simulink model "node23_case_10kV_withLoad_v2"  (R2022b)
settings: Solver=VariableStepAuto  StartTime=0.0  StopTime=10  FixedStep=1e-6  RelTol=1e-5
InitFcn:
  | sw=5;
  | Lf=1.75e-3+3.5e-3;
  | %Lf=3.5e-3;
  | %Cf=2e-4;
  | f=10;
  | Cf=15e-6;
  | % L=1.75e-3/2;
  | % X=100*pi*L;
  | % R=2*X;
  | R=0.25;X=R/0.66;
  | L=X/100/pi;
  | Z=sqrt(R^2+X^2);
  | f = 30;
  | kp1=10;
  | ki1=100;
  | kp4=20;
  | ki4=100;
  | kp16=20;
  | ki16=100;
  | % 负载参数
  | R1L=0;
  | X1L=0;
  | R2L=652.4467;
  | X2L=276.0351;
  | R3L=804.5741;
  | X3L=256.7790;
  | R4L=760.9867;
  | X4L=234.6376;
  | R5L=818.7384;
  | X5L=266.9799;
  | R6L=671.1329;
  | X6L=170.1801;
  | R7L=883.7621;
  | X7L=178.8663;
  | R8L=388.3725;
  | X8L=158.3040;
  | R9L=817.4819;
  | X9L=268.6933;
  | R10L=849.4733;
  | X10L=254.8420;
  | R11L=407.8415;
  | X11L=165.8504;
  | R12L=NaN;  % Bus 12 无 R、X 数据，用 NaN 标记
  | X12L=NaN;
  | R13L=751.2339;
  | X13L=329.8428;
  | R14L=294.0393;
  | X14L=141.6929;
  | R15L=761.9027;
  | X15L=284.3908;
  | R16L=740.4040;
  | X16L=318.2438;
  | R17L=674.5784;
  | X17L=316.4689;
  | R18L=776.7449;
  | X18L=316.6080;
  | R19L=766.0423;
  | X19L=335.7994;
  | R20L=746.0545;
  | X20L=344.3329;
  | R21L=706.9418;
  | X21L=357.8658;
  | R22L=702.3905;
  | X22L=304.8773;
  | R23L=244.5696;
  | X23L=118.4449;
  | %% Case 1
  | % I4dp_ref = 68.7653;
  | % I4qp_ref = -94.1021;
  | % I4dn_ref = 39.6776;
  | % I4qn_ref = -27.1728;
  | % I8dp_ref = 68.5903;
  | % I8qp_ref = -93.5945;
  | % I8dn_ref = 40.6189;
  | % I8qn_ref = -26.6634;
  | % I10dp_ref = 62.5266;
  | % I10qp_ref = -85.5137;
  | % I10dn_ref = 42.9996;
  | % I10qn_ref = -28.7612;
  | % I11dp_ref = 62.7521;
  | % I11qp_ref = -85.7827;
  | % I11dn_ref = 42.8345;
  | % I11qn_ref = -28.6532;
  | % I12dp_ref = 62.3475;
  | % I12qp_ref = -85.2997;
  | % I12dn_ref = 43.1344;
  | % I12qn_ref = -28.848;
  | % I16dp_ref = 82.4934;
  | % I16qp_ref = -110.4734;
  | % I16dn_ref = 40.1418;
  | % I16qn_ref = -24.7044;
  | % I21dp_ref = 73.1603;
  | % I21qp_ref = -97.1416;
  | % I21dn_ref = 45.9939;
  | % I21qn_ref = -31.0997;
  | % I22dp_ref = 80.0535;
  | % I22qp_ref = -107.1896;
  | % I22dn_ref = 40.9482;
  | % I22qn_ref = -26.0625;
  | % I23dp_ref = 75.9498;
  | % I23qp_ref = -101.1053;
  | % I23dn_ref = 43.7688;
  | % I23qn_ref = -29.0712;
  | %% Case1 comparison 1
  | % I4dp_ref = 111.7874;
  | % I4qp_ref = -170.7915;
  | % I4dn_ref = 0;
  | % I4qn_ref = 0;
  | % I8dp_ref = 52.2536;
  | % I8qp_ref = -33.9901;
  | % I8dn_ref = 0;
  | % I8qn_ref = 0;
  | % I10dp_ref = 33.1037;
  | % I10qp_ref = -19.0499;
  | % I10dn_ref = 0;
  | % I10qn_ref = 0;
  | % I11dp_ref = 43.6215;
  | % I11qp_ref = -22.5412;
  | % I11dn_ref = 0;
  | % I11qn_ref = 0;
  | % I12dp_ref = 8.2667;
  | % I12qp_ref = -27.5019;
  | % I12dn_ref = 0;
  | % I12qn_ref = 0;
  | % I16dp_ref = 104.5239;
  | % I16qp_ref = -104.5004;
  | % I16dn_ref = 0;
  | % I16qn_ref = 0;
  | % I21dp_ref = 68.3072;
  | % I21qp_ref = 6.327;
  | % I21dn_ref = 0;
  | % I21qn_ref = 0;
  | % I22dp_ref = 124.4645;
  | % I22qp_ref = -71.238;
  | % I22dn_ref = 0;
  | % I22qn_ref = 0;
  | % I23dp_ref = -36.8953;
  | % I23qp_ref = -101.2509;
  | % I23dn_ref = 0;
  | % I23qn_ref = 0;
  | 
  | % %%case 1 S2
  | % I4dp_ref = 0;
  | % I4qp_ref = 0;
  | % I4dn_ref = 42.8306;
  | % I4qn_ref = 0;
  | % I8dp_ref = 0;
  | % I8qp_ref = 0;
  | % I8dn_ref = 0;
  | % I8qn_ref = -148.8111;
  | % I10dp_ref = 0;
  | % I10qp_ref = 0;
  | % I10dn_ref = 204.1241;
  | % I10qn_ref = 0;
  | % I11dp_ref = 0;
  | % I11qp_ref = 0;
  | % I11dn_ref = 0;
  | % I11qn_ref = -7.0259;
  | % I12dp_ref = 0;
  | % I12qp_ref = 0;
  | % I12dn_ref = 59.8066;
  | % I12qn_ref = 0;
  | % I16dp_ref = 0;
  | % I16qp_ref = 0;
  | % I16dn_ref = 0;
  | % I16qn_ref = 40.0795;
  | % I21dp_ref = 0;
  | % I21qp_ref = 0;
  | % I21dn_ref = 133.7305;
  | % I21qn_ref = 41.6572;
  | % I22dp_ref = 0;
  | % I22qp_ref = 0;
  | % I22dn_ref = 0;
  | % I22qn_ref = 0;
  | % I23dp_ref = 0;
  | % I23qp_ref = 0;
  | % I23dn_ref = 0;
  | % I23qn_ref = -141.9369;
  | %% Case 2
  | % I4dp_ref = 59.2929;
  | % I4qp_ref = -107.5927;
  | % I4dn_ref = -11.6305;
  | % I4qn_ref = -80.5926;
  | % I8dp_ref = 59.4332;
  | % I8qp_ref = -112.5957;
  | % I8dn_ref = -13.993;
  | % I8qn_ref = -80.1364;
  | % I10dp_ref = 58.9639;
  | % I10qp_ref = -112.9937;
  | % I10dn_ref = -14.0895;
  | % I10qn_ref = -80.4774;
  | % I11dp_ref = 59.0086;
  | % I11qp_ref = -112.9917;
  | % I11dn_ref = -14.1006;
  | % I11qn_ref = -80.4455;
  | % I12dp_ref = 58.9134;
  | % I12qp_ref = -112.9993;
  | % I12dn_ref = -14.0713;
  | % I12qn_ref = -80.5073;
  | % I16dp_ref = 60.7969;
  | % I16qp_ref = -109.8449;
  | % I16dn_ref = -12.6646;
  | % I16qn_ref = -78.7002;
  | % I21dp_ref = 61.3666;
  | % I21qp_ref = -114.9373;
  | % I21dn_ref = -14.6537;
  | % I21qn_ref = -77.5067;
  | % I22dp_ref = 61.0222;
  | % I22qp_ref = -111.4137;
  | % I22dn_ref = -13.2536;
  | % I22qn_ref = -78.3425;
  | % I23dp_ref = 61.4875;
  | % I23qp_ref = -114.3173;
  | % I23dn_ref = -14.4491;
  | % I23qn_ref = -77.5307;
  | 
  | %% case 2 S1
  | % I4dp_ref = 112.192;
  | % I4qp_ref = -170.5275;
  | % I4dn_ref = 0;
  | % I4qn_ref = 0;
  | % I8dp_ref = 112.2722;
  | % I8qp_ref = -170.4747;
  | % I8dn_ref = 0;
  | % I8qn_ref = 0;
  | % I10dp_ref = 111.9451;
  | % I10qp_ref = -170.6897;
  | % I10dn_ref = 0;
  | % I10qn_ref = 0;
  | % I11dp_ref = 111.9882;
  | % I11qp_ref = -170.6614;
  | % I11dn_ref = 0;
  | % I11qn_ref = 0;
  | % I12dp_ref = 111.8926;
  | % I12qp_ref = -170.7241;
  | % I12dn_ref = 0;
  | % I12qn_ref = 0;
  | % I16dp_ref = 112.3621;
  | % I16qp_ref = -170.4154;
  | % I16dn_ref = 0;
  | % I16qn_ref = 0;
  | % I21dp_ref = 112.3273;
  | % I21qp_ref = -170.4384;
  | % I21dn_ref = 0;
  | % I21qn_ref = 0;
  | % I22dp_ref = 112.3902;
  | % I22qp_ref = -170.3969;
  | % I22dn_ref = 0;
  | % I22qn_ref = 0;
  | % I23dp_ref = 112.4817;
  | % I23qp_ref = -170.3365;
  | % I23dn_ref = 0;
  | % I23qn_ref = 0;
  | %% case 2 S2
  | % I4dp_ref = 0;
  | % I4qp_ref = 0;
  | % I4dn_ref = 69.83;
  | % I4qn_ref = -191.8084;
  | % I8dp_ref = 0;
  | % I8qp_ref = 0;
  | % I8dn_ref = -20.269;
  | % I8qn_ref = -203.1153;
  | % I10dp_ref = 0;
  | % I10qp_ref = 0;
  | % I10dn_ref = -45.3511;
  | % I10qn_ref = -199.0225;
  | % I11dp_ref = 0;
  | % I11qp_ref = 0;
  | % I11dn_ref = -12.4369;
  | % I11qn_ref = -203.7449;
  | % I12dp_ref = 0;
  | % I12qp_ref = 0;
  | % I12dn_ref = -12.1733;
  | % I12qn_ref = -203.7608;
  | % I16dp_ref = 0;
  | % I16qp_ref = 0;
  | % I16dn_ref = 48.8908;
  | % I16qn_ref = -198.1826;
  | % I21dp_ref = 0;
  | % I21qp_ref = 0;
  | % I21dn_ref = -43.073;
  | % I21qn_ref = -199.5279;
  | % I22dp_ref = 0;
  | % I22qp_ref = 0;
  | % I22dn_ref = 39.4057;
  | % I22qn_ref = -200.2844;
  | % I23dp_ref = 0;
  | % I23qp_ref = 0;
  | % I23dn_ref = -19.2428;
  | % I23qn_ref = -203.2151;
  | I4dp_ref = 0.9372;
  | I4qp_ref = -0.47047;
  | I4dn_ref = 170.1426;
  | I4qn_ref = -111.8156;
  | I8dp_ref = 28.4579;
  | I8qp_ref = -127.0294;
  | I8dn_ref = 23.3009;
  | I8qn_ref = -14.8212;
  | I10dp_ref = 27.4288;
  | I10qp_ref = -127.8154;
  | I10dn_ref = 16.0506;
  | I10qn_ref = -10.7004;
  | I11dp_ref = 27.4818;
  | I11qp_ref = -127.8231;
  | I11dn_ref = 15.959;
  | I11qn_ref = -10.8247;
  | I12dp_ref = 27.4417;
  | I12qp_ref = -127.7991;
  | I12dn_ref = 16.0832;
  | I12qn_ref = -10.7612;
  | I16dp_ref = 30.7964;
  | I16qp_ref = -47.2674;
  | I16dn_ref = 97.2786;
  | I16qn_ref = -63.7105;
  | I21dp_ref = 33.4859;
  | I21qp_ref = -81.6358;
  | I21dn_ref = 15.3458;
  | I21qn_ref = -5.5591;
  | I22dp_ref = 31.8848;
  | I22qp_ref = -57.1916;
  | I22dn_ref = 83.6176;
  | I22qn_ref = -53.4829;
  | I23dp_ref = 33.8327;
  | I23qp_ref = -82.3263;
  | I23dn_ref = 11.5111;
  | I23qn_ref = -14.1008;
libraries: spsSeriesRLCBranchLib x210, slpidlib x45, spsControlledVoltageSourceLib x30, spsThreePhaseVIMeasurementLib x24, spsPower3phInstantaneousLib x13, spsAlphaBetaZerotoabcLib x9, spsCurrentMeasurementLib x6, spsGroundLib x2, spspowerguiLib x1
(part 1 of 8)
settings Model: SimulationMode=rapid-accelerator  Creator=15224  LastModifiedBy=Sweet_J
settings SolverCC: AlgebraicLoopSolver=TrustRegion
settings DataIOCC: ReturnWorkspaceOutputs=off
settings DebuggingCC: UnconnectedInputMsg=warning  UnconnectedOutputMsg=warning  UnconnectedLineMsg=warning  SFMachineParentedDataDiag=warning  ArithmeticOperatorsInVariantConditions=warning
settings ModelReferenceCC: EnableRefExpFcnMdlSchedulingChecks=on
settings SFSimCC: CustomCodeUndefinedFunction=UseInterfaceOnly

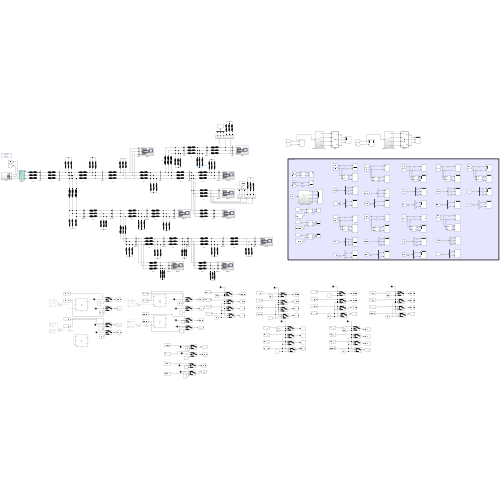
[thumbnail: Simulink's stored preview of the top-level diagram]
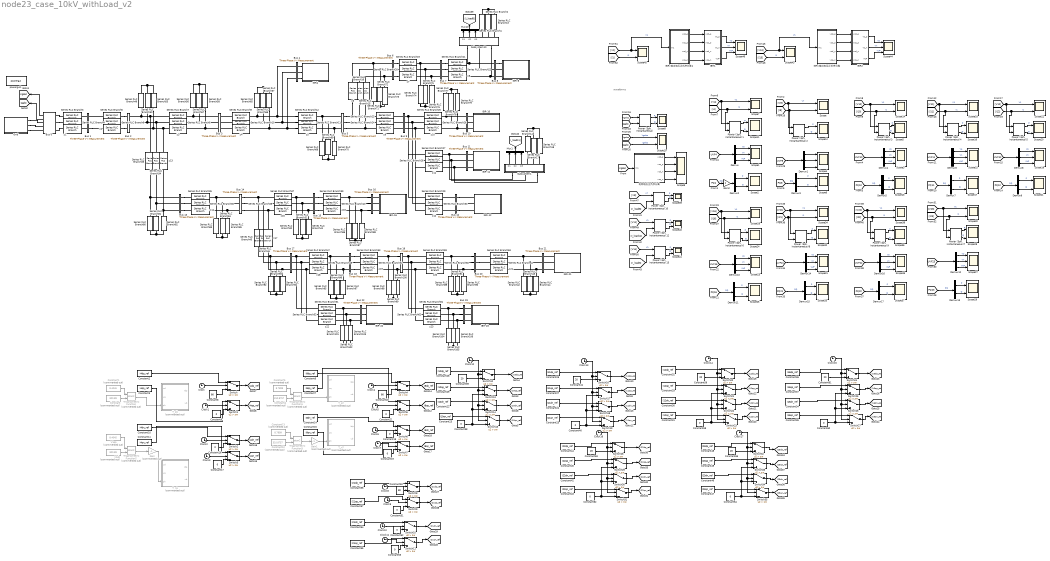
== system node23_case_10kV_withLoad_v2 ==
  note: waveforms
  Bus 0 : spsThreePhaseVIMeasurementLib/Three-Phase V-I Measurement  VoltageMeasurement=phase-to-ground  SetLabelV=off  LabelV=Vabc  Vpu=off  VpuLL=off  CurrentMeasurement=yes  SetLabelI=off  LabelI=Iabc  Ipu=off  Pbase=100e6  Vbase=500e3  OutputType=Complex  PhasorSimulation=off  PSBequivalent=0
  Bus 1 : spsThreePhaseVIMeasurementLib/Three-Phase V-I Measurement  VoltageMeasurement=phase-to-ground  SetLabelV=on  LabelV=V1  Vpu=off  VpuLL=off  CurrentMeasurement=yes  SetLabelI=on  LabelI=I1  Ipu=off  Pbase=100e6  Vbase=500e3  OutputType=Complex  PhasorSimulation=off  PSBequivalent=0
  Bus 10 : spsThreePhaseVIMeasurementLib/Three-Phase V-I Measurement  VoltageMeasurement=phase-to-ground  SetLabelV=on  LabelV=V10  Vpu=off  VpuLL=off  CurrentMeasurement=yes  SetLabelI=on  LabelI=I10  Ipu=off  Pbase=100e6  Vbase=500e3  OutputType=Complex  PhasorSimulation=off  PSBequivalent=0
  Bus 11 : spsThreePhaseVIMeasurementLib/Three-Phase V-I Measurement  VoltageMeasurement=phase-to-ground  SetLabelV=on  LabelV=V11  Vpu=off  VpuLL=off  CurrentMeasurement=yes  SetLabelI=on  LabelI=I11  Ipu=off  Pbase=100e6  Vbase=500e3  OutputType=Complex  PhasorSimulation=off  PSBequivalent=0
  Bus 12 : spsThreePhaseVIMeasurementLib/Three-Phase V-I Measurement  VoltageMeasurement=phase-to-ground  SetLabelV=on  LabelV=V12  Vpu=off  VpuLL=off  CurrentMeasurement=yes  SetLabelI=on  LabelI=I12  Ipu=off  Pbase=100e6  Vbase=500e3  OutputType=Complex  PhasorSimulation=off  PSBequivalent=0
  Bus 13 : spsThreePhaseVIMeasurementLib/Three-Phase V-I Measurement  VoltageMeasurement=phase-to-ground  SetLabelV=on  LabelV=V13  Vpu=off  VpuLL=off  CurrentMeasurement=yes  SetLabelI=on  LabelI=I13  Ipu=off  Pbase=100e6  Vbase=500e3  OutputType=Complex  PhasorSimulation=off  PSBequivalent=0
  Bus 14 : spsThreePhaseVIMeasurementLib/Three-Phase V-I Measurement  VoltageMeasurement=phase-to-ground  SetLabelV=on  LabelV=V14  Vpu=off  VpuLL=off  CurrentMeasurement=yes  SetLabelI=on  LabelI=I14  Ipu=off  Pbase=100e6  Vbase=500e3  OutputType=Complex  PhasorSimulation=off  PSBequivalent=0
  Bus 15 : spsThreePhaseVIMeasurementLib/Three-Phase V-I Measurement  VoltageMeasurement=phase-to-ground  SetLabelV=on  LabelV=V15  Vpu=off  VpuLL=off  CurrentMeasurement=yes  SetLabelI=on  LabelI=I15  Ipu=off  Pbase=100e6  Vbase=500e3  OutputType=Complex  PhasorSimulation=off  PSBequivalent=0
  Bus 16 : spsThreePhaseVIMeasurementLib/Three-Phase V-I Measurement  VoltageMeasurement=phase-to-ground  SetLabelV=on  LabelV=V16  Vpu=off  VpuLL=off  CurrentMeasurement=yes  SetLabelI=on  LabelI=I16  Ipu=off  Pbase=100e6  Vbase=500e3  OutputType=Complex  PhasorSimulation=off  PSBequivalent=0
  Bus 17 : spsThreePhaseVIMeasurementLib/Three-Phase V-I Measurement  VoltageMeasurement=phase-to-ground  SetLabelV=on  LabelV=V17  Vpu=off  VpuLL=off  CurrentMeasurement=yes  SetLabelI=on  LabelI=I17  Ipu=off  Pbase=100e6  Vbase=500e3  OutputType=Complex  PhasorSimulation=off  PSBequivalent=0
  Bus 18 : spsThreePhaseVIMeasurementLib/Three-Phase V-I Measurement  VoltageMeasurement=phase-to-ground  SetLabelV=on  LabelV=V18  Vpu=off  VpuLL=off  CurrentMeasurement=yes  SetLabelI=on  LabelI=I18  Ipu=off  Pbase=100e6  Vbase=500e3  OutputType=Complex  PhasorSimulation=off  PSBequivalent=0
  Bus 19 : spsThreePhaseVIMeasurementLib/Three-Phase V-I Measurement  VoltageMeasurement=phase-to-ground  SetLabelV=on  LabelV=V19  Vpu=off  VpuLL=off  CurrentMeasurement=yes  SetLabelI=on  LabelI=I19  Ipu=off  Pbase=100e6  Vbase=500e3  OutputType=Complex  PhasorSimulation=off  PSBequivalent=0
  Bus 2 : spsThreePhaseVIMeasurementLib/Three-Phase V-I Measurement  VoltageMeasurement=phase-to-ground  SetLabelV=on  LabelV=V2  Vpu=off  VpuLL=off  CurrentMeasurement=yes  SetLabelI=on  LabelI=I2  Ipu=off  Pbase=100e6  Vbase=500e3  OutputType=Complex  PhasorSimulation=off  PSBequivalent=0
  Bus 20 : spsThreePhaseVIMeasurementLib/Three-Phase V-I Measurement  VoltageMeasurement=phase-to-ground  SetLabelV=on  LabelV=V20  Vpu=off  VpuLL=off  CurrentMeasurement=yes  SetLabelI=on  LabelI=I20  Ipu=off  Pbase=100e6  Vbase=500e3  OutputType=Complex  PhasorSimulation=off  PSBequivalent=0
  Bus 21 : spsThreePhaseVIMeasurementLib/Three-Phase V-I Measurement  VoltageMeasurement=phase-to-ground  SetLabelV=on  LabelV=V21  Vpu=off  VpuLL=off  CurrentMeasurement=yes  SetLabelI=on  LabelI=I21  Ipu=off  Pbase=100e6  Vbase=500e3  OutputType=Complex  PhasorSimulation=off  PSBequivalent=0
  Bus 22 : spsThreePhaseVIMeasurementLib/Three-Phase V-I Measurement  VoltageMeasurement=phase-to-ground  SetLabelV=on  LabelV=V22  Vpu=off  VpuLL=off  CurrentMeasurement=yes  SetLabelI=on  LabelI=I22  Ipu=off  Pbase=100e6  Vbase=500e3  OutputType=Complex  PhasorSimulation=off  PSBequivalent=0
  Bus 23 : spsThreePhaseVIMeasurementLib/Three-Phase V-I Measurement  VoltageMeasurement=phase-to-ground  SetLabelV=on  LabelV=V23  Vpu=off  VpuLL=off  CurrentMeasurement=yes  SetLabelI=on  LabelI=I23  Ipu=off  Pbase=100e6  Vbase=500e3  OutputType=Complex  PhasorSimulation=off  PSBequivalent=0
  Bus 3 : spsThreePhaseVIMeasurementLib/Three-Phase V-I Measurement  VoltageMeasurement=phase-to-ground  SetLabelV=on  LabelV=V3  Vpu=off  VpuLL=off  CurrentMeasurement=yes  SetLabelI=on  LabelI=I3  Ipu=off  Pbase=100e6  Vbase=500e3  OutputType=Complex  PhasorSimulation=off  PSBequivalent=0
  Bus 4 : spsThreePhaseVIMeasurementLib/Three-Phase V-I Measurement  VoltageMeasurement=phase-to-ground  SetLabelV=on  LabelV=V4  Vpu=off  VpuLL=off  CurrentMeasurement=yes  SetLabelI=on  LabelI=I4  Ipu=off  Pbase=100e6  Vbase=500e3  OutputType=Complex  PhasorSimulation=off  PSBequivalent=0
  Bus 5 : spsThreePhaseVIMeasurementLib/Three-Phase V-I Measurement  VoltageMeasurement=phase-to-ground  SetLabelV=on  LabelV=V5  Vpu=off  VpuLL=off  CurrentMeasurement=yes  SetLabelI=on  LabelI=I5  Ipu=off  Pbase=100e6  Vbase=500e3  OutputType=Complex  PhasorSimulation=off  PSBequivalent=0
  Bus 6 : spsThreePhaseVIMeasurementLib/Three-Phase V-I Measurement  VoltageMeasurement=phase-to-ground  SetLabelV=on  LabelV=V6  Vpu=off  VpuLL=off  CurrentMeasurement=yes  SetLabelI=on  LabelI=I6  Ipu=off  Pbase=100e6  Vbase=500e3  OutputType=Complex  PhasorSimulation=off  PSBequivalent=0
  Bus 7 : spsThreePhaseVIMeasurementLib/Three-Phase V-I Measurement  VoltageMeasurement=phase-to-ground  SetLabelV=on  LabelV=V7  Vpu=off  VpuLL=off  CurrentMeasurement=yes  SetLabelI=on  LabelI=I7  Ipu=off  Pbase=100e6  Vbase=500e3  OutputType=Complex  PhasorSimulation=off  PSBequivalent=0
  Bus 8 : spsThreePhaseVIMeasurementLib/Three-Phase V-I Measurement  VoltageMeasurement=phase-to-ground  SetLabelV=on  LabelV=V8  Vpu=off  VpuLL=off  CurrentMeasurement=yes  SetLabelI=on  LabelI=I8  Ipu=off  Pbase=100e6  Vbase=500e3  OutputType=Complex  PhasorSimulation=off  PSBequivalent=0
  Bus 9 : spsThreePhaseVIMeasurementLib/Three-Phase V-I Measurement  VoltageMeasurement=phase-to-ground  SetLabelV=on  LabelV=V9  Vpu=off  VpuLL=off  CurrentMeasurement=yes  SetLabelI=on  LabelI=I9  Ipu=off  Pbase=100e6  Vbase=500e3  OutputType=Complex  PhasorSimulation=off  PSBequivalent=0
  Clock{,1..17} (18 alike) : Clock
  Constant : Constant  Commented=on  Value=300.89
  Constant1 : Constant  Commented=on  Value=8.4045
  Constant10 : Constant  Value=I4dn_ref
  Constant11 : Constant  Value=I4qn_ref
  Constant12 : Constant  Commented=on  Value=310.8757
  Constant13 : Constant  Commented=on  Value=8.7899
  Constant14 : Constant  Value=I8dn_ref
  Constant15 : Constant  Value=I8qn_ref
  Constant{9,16..19,21,38,40,51..53,58,60,62,64} (15 alike) : Constant  Value=0
  Constant2 : Constant  Value=I4dp_ref
  Constant20 : Constant  Value=80
  Constant22 : Constant  Value=I10dn_ref
  Constant23 : Constant  Value=I10qn_ref
  Constant24 : Constant  Value=I11dn_ref
  Constant25 : Constant  Value=I11qn_ref
  Constant26 : Constant  Value=I11dp_ref
  Constant27 : Constant  Value=I11qp_ref
  Constant28 : Constant  Value=I10dp_ref
  Constant29 : Constant  Value=I10qp_ref
  Constant3 : Constant  Value=I4qp_ref
  Constant30 : Constant  Value=I12dn_ref
  Constant31 : Constant  Value=I12qn_ref
  Constant32 : Constant  Value=I12dp_ref
  Constant33 : Constant  Value=I12qp_ref
  Constant34 : Constant  Value=I16dn_ref
  Constant35 : Constant  Value=I16qn_ref
  Constant36 : Constant  Value=I16dp_ref
  Constant37 : Constant  Value=I16qp_ref
  Constant{39,41,59,61,63,65} (6 alike) : Constant  Value=20
  Constant4 : Constant  Commented=on  Value=310.8757
  Constant42 : Constant  Value=I22dn_ref
  Constant43 : Constant  Value=I22qn_ref
  Constant44 : Constant  Value=I22dp_ref
  Constant45 : Constant  Value=I22qp_ref
  Constant46 : Constant  Value=I23dn_ref
  Constant47 : Constant  Value=I23qn_ref
  Constant48 : Constant  Value=I23dp_ref
  Constant49 : Constant  Value=I23qp_ref
  Constant5 : Constant  Commented=on  Value=8.7899
  Constant50 : Constant  Value=80
  Constant54 : Constant  Value=I21dn_ref
  Constant55 : Constant  Value=I21qn_ref
  Constant56 : Constant  Value=I21dp_ref
  Constant57 : Constant  Value=I21qp_ref
  Constant6 : Constant  Value=I8dp_ref
  Constant7 : Constant  Value=I8qp_ref
  Constant8 : Constant  Value=80
  Demux{,1,4,6,8,10,12,14,16} (9 alike) : Demux  Outputs=3
  Demux{2..3,5,7,9,11,13,15,17} (9 alike) : Demux  Outputs=2
  Gain : Gain  Commented=on  Gain=-1
  Gain1 : Gain  Commented=on  Gain=-1
  Gain2 : Gain
  Grid : Subsystem
  IBR-10 : Subsystem
  IBR-11 : Subsystem
  IBR-12 : Subsystem
  IBR-16 : Subsystem
  IBR-21 : Subsystem
  IBR-22 : Subsystem
  IBR-23 : Subsystem
  IBR-8 : Subsystem
  IBR1 : MATLAB Function  TreatAsAtomicUnit=on
  IBR1输出电压正负序分离 : Subsystem
  IBR1输出电压正负序分离1 : Subsystem
  IBR2 : MATLAB Function  TreatAsAtomicUnit=on
  IBR4 : Subsystem
  Mux1 : Mux  Inputs=3
  Mux10 : Mux  Inputs=3
  Power (3ph, Instantaneous){,1..10,12..13} (13 alike) : spsPower3phInstantaneousLib/Power (3ph, Instantaneous)
  Scope{,2,5..8,10..14,16..18,20..22,24..26,28..30,32..34,36..41,43,45} (34 alike) : Scope  NumInputPorts=2
  Scope{1,3..4,15,19,23,27,31,35,44,46} (11 alike) : Scope  NumInputPorts=3
  Scope9 : Scope  NumInputPorts=4
  Series RLC Branch1 : spsSeriesRLCBranchLib/Series RLC Branch  LConnTagsString=__new0  RConnTagsString=__new0  BranchType=RL  Resistance=R8L  Inductance=X8L/100/pi  SetiL0=off  InitialCurrent=0  Capacitance=1e-6  Setx0=off  InitialVoltage=0  Measurements=None
  Series RLC Branch{3..12,15..16,19..30,33..40,45..48,51..54,59..64} (46 alike) : spsSeriesRLCBranchLib/Series RLC Branch  LConnTagsString=__new0  RConnTagsString=__new0  BranchType=RL  Resistance=R  Inductance=L  SetiL0=off  InitialCurrent=0  Capacitance=1e-6  Setx0=off  InitialVoltage=0  Measurements=None
  Series RLC Branch100 : spsSeriesRLCBranchLib/Series RLC Branch  LConnTagsString=__new0  RConnTagsString=__new0  BranchType=RL  Resistance=R19L  Inductance=X19L/100/pi  SetiL0=off  InitialCurrent=0  Capacitance=1e-6  Setx0=off  InitialVoltage=0  Measurements=None
  Series RLC Branch101 : spsSeriesRLCBranchLib/Series RLC Branch  LConnTagsString=__new0  RConnTagsString=__new0  BranchType=RL  Resistance=R22L  Inductance=X22L/100/pi  SetiL0=off  InitialCurrent=0  Capacitance=1e-6  Setx0=off  InitialVoltage=0  Measurements=None
  Series RLC Branch102 : spsSeriesRLCBranchLib/Series RLC Branch  LConnTagsString=__new0  RConnTagsString=__new0  BranchType=RL  Resistance=R22L  Inductance=X22L/100/pi  SetiL0=off  InitialCurrent=0  Capacitance=1e-6  Setx0=off  InitialVoltage=0  Measurements=None
  Series RLC Branch103 : spsSeriesRLCBranchLib/Series RLC Branch  LConnTagsString=__new0  RConnTagsString=__new0  BranchType=RL  Resistance=R22L  Inductance=X22L/100/pi  SetiL0=off  InitialCurrent=0  Capacitance=1e-6  Setx0=off  InitialVoltage=0  Measurements=None
  Series RLC Branch104 : spsSeriesRLCBranchLib/Series RLC Branch  LConnTagsString=__new0  RConnTagsString=__new0  BranchType=RL  Resistance=R23L  Inductance=X23L/100/pi  SetiL0=off  InitialCurrent=0  Capacitance=1e-6  Setx0=off  InitialVoltage=0  Measurements=None
  Series RLC Branch105 : spsSeriesRLCBranchLib/Series RLC Branch  LConnTagsString=__new0  RConnTagsString=__new0  BranchType=RL  Resistance=R23L  Inductance=X23L/100/pi  SetiL0=off  InitialCurrent=0  Capacitance=1e-6  Setx0=off  InitialVoltage=0  Measurements=None
  Series RLC Branch106 : spsSeriesRLCBranchLib/Series RLC Branch  LConnTagsString=__new0  RConnTagsString=__new0  BranchType=RL  Resistance=R23L  Inductance=X23L/100/pi  SetiL0=off  InitialCurrent=0  Capacitance=1e-6  Setx0=off  InitialVoltage=0  Measurements=None
  Series RLC Branch13 : spsSeriesRLCBranchLib/Series RLC Branch  LConnTagsString=__new0  RConnTagsString=__new0  BranchType=RL  Resistance=R8L  Inductance=X8L/100/pi  SetiL0=off  InitialCurrent=0  Capacitance=1e-6  Setx0=off  InitialVoltage=0  Measurements=None
  Series RLC Branch14 : spsSeriesRLCBranchLib/Series RLC Branch  LConnTagsString=__new0  RConnTagsString=__new0  BranchType=RL  Resistance=R11L  Inductance=X11L/100/pi  SetiL0=off  InitialCurrent=0  Capacitance=1e-6  Setx0=off  InitialVoltage=0  Measurements=None
  Series RLC Branch17 : spsSeriesRLCBranchLib/Series RLC Branch  LConnTagsString=__new0  RConnTagsString=__new0  BranchType=RL  Resistance=R11L  Inductance=X11L/100/pi  SetiL0=off  InitialCurrent=0  Capacitance=1e-6  Setx0=off  InitialVoltage=0  Measurements=None
  Series RLC Branch18 : spsSeriesRLCBranchLib/Series RLC Branch  LConnTagsString=__new0  RConnTagsString=__new0  BranchType=RL  Resistance=R11L  Inductance=X11L/100/pi  SetiL0=off  InitialCurrent=0  Capacitance=1e-6  Setx0=off  InitialVoltage=0  Measurements=None
  Series RLC Branch2 : spsSeriesRLCBranchLib/Series RLC Branch  LConnTagsString=__new0  RConnTagsString=__new0  BranchType=RL  Resistance=R8L  Inductance=X8L/100/pi  SetiL0=off  InitialCurrent=0  Capacitance=1e-6  Setx0=off  InitialVoltage=0  Measurements=None
  Series RLC Branch31 : spsSeriesRLCBranchLib/Series RLC Branch  LConnTagsString=__new0  RConnTagsString=__new0  BranchType=RL  Resistance=R15L  Inductance=X15L/100/pi  SetiL0=off  InitialCurrent=0  Capacitance=1e-6  Setx0=off  InitialVoltage=0  Measurements=None
  Series RLC Branch32 : spsSeriesRLCBranchLib/Series RLC Branch  LConnTagsString=__new0  RConnTagsString=__new0  BranchType=RL  Resistance=R15L  Inductance=X15L/100/pi  SetiL0=off  InitialCurrent=0  Capacitance=1e-6  Setx0=off  InitialVoltage=0  Measurements=None
  Series RLC Branch41 : spsSeriesRLCBranchLib/Series RLC Branch  LConnTagsString=__new0  RConnTagsString=__new0  BranchType=RL  Resistance=R15L  Inductance=X15L/100/pi  SetiL0=off  InitialCurrent=0  Capacitance=1e-6  Setx0=off  InitialVoltage=0  Measurements=None
  Series RLC Branch42 : spsSeriesRLCBranchLib/Series RLC Branch  LConnTagsString=__new0  RConnTagsString=__new0  BranchType=RL  Resistance=R21L  Inductance=X21L/100/pi  SetiL0=off  InitialCurrent=0  Capacitance=1e-6  Setx0=off  InitialVoltage=0  Measurements=None
  Series RLC Branch43 : spsSeriesRLCBranchLib/Series RLC Branch  LConnTagsString=__new0  RConnTagsString=__new0  BranchType=RL  Resistance=R21L  Inductance=X21L/100/pi  SetiL0=off  InitialCurrent=0  Capacitance=1e-6  Setx0=off  InitialVoltage=0  Measurements=None
  Series RLC Branch44 : spsSeriesRLCBranchLib/Series RLC Branch  LConnTagsString=__new0  RConnTagsString=__new0  BranchType=RL  Resistance=R21L  Inductance=X21L/100/pi  SetiL0=off  InitialCurrent=0  Capacitance=1e-6  Setx0=off  InitialVoltage=0  Measurements=None
  Series RLC Branch49 : spsSeriesRLCBranchLib/Series RLC Branch  LConnTagsString=__new0  RConnTagsString=__new0  BranchType=RL  Resistance=R2L  Inductance=X2L/100/pi  SetiL0=off  InitialCurrent=0  Capacitance=1e-6  Setx0=off  InitialVoltage=0  Measurements=None
  Series RLC Branch50 : spsSeriesRLCBranchLib/Series RLC Branch  LConnTagsString=__new0  RConnTagsString=__new0  BranchType=RL  Resistance=R2L  Inductance=X2L/100/pi  SetiL0=off  InitialCurrent=0  Capacitance=1e-6  Setx0=off  InitialVoltage=0  Measurements=None
  Series RLC Branch55 : spsSeriesRLCBranchLib/Series RLC Branch  LConnTagsString=__new0  RConnTagsString=__new0  BranchType=RL  Resistance=R2L  Inductance=X2L/100/pi  SetiL0=off  InitialCurrent=0  Capacitance=1e-6  Setx0=off  InitialVoltage=0  Measurements=None
  Series RLC Branch56 : spsSeriesRLCBranchLib/Series RLC Branch  LConnTagsString=__new0  RConnTagsString=__new0  BranchType=RL  Resistance=R3L  Inductance=X3L/100/pi  SetiL0=off  InitialCurrent=0  Capacitance=1e-6  Setx0=off  InitialVoltage=0  Measurements=None
  Series RLC Branch57 : spsSeriesRLCBranchLib/Series RLC Branch  LConnTagsString=__new0  RConnTagsString=__new0  BranchType=RL  Resistance=R3L  Inductance=X3L/100/pi  SetiL0=off  InitialCurrent=0  Capacitance=1e-6  Setx0=off  InitialVoltage=0  Measurements=None
  Series RLC Branch58 : spsSeriesRLCBranchLib/Series RLC Branch  LConnTagsString=__new0  RConnTagsString=__new0  BranchType=RL  Resistance=R3L  Inductance=X3L/100/pi  SetiL0=off  InitialCurrent=0  Capacitance=1e-6  Setx0=off  InitialVoltage=0  Measurements=None
  Series RLC Branch65 : spsSeriesRLCBranchLib/Series RLC Branch  LConnTagsString=__new0  RConnTagsString=__new0  BranchType=RL  Resistance=R4L  Inductance=X4L/100/pi  SetiL0=off  InitialCurrent=0  Capacitance=1e-6  Setx0=off  InitialVoltage=0  Measurements=None
  Series RLC Branch66 : spsSeriesRLCBranchLib/Series RLC Branch  LConnTagsString=__new0  RConnTagsString=__new0  BranchType=RL  Resistance=R4L  Inductance=X4L/100/pi  SetiL0=off  InitialCurrent=0  Capacitance=1e-6  Setx0=off  InitialVoltage=0  Measurements=None
  Series RLC Branch67 : spsSeriesRLCBranchLib/Series RLC Branch  LConnTagsString=__new0  RConnTagsString=__new0  BranchType=RL  Resistance=R4L  Inductance=X4L/100/pi  SetiL0=off  InitialCurrent=0  Capacitance=1e-6  Setx0=off  InitialVoltage=0  Measurements=None
  Series RLC Branch68 : spsSeriesRLCBranchLib/Series RLC Branch  LConnTagsString=__new0  RConnTagsString=__new0  BranchType=RL  Resistance=R5L  Inductance=X5L/100/pi  SetiL0=off  InitialCurrent=0  Capacitance=1e-6  Setx0=off  InitialVoltage=0  Measurements=None
  Series RLC Branch69 : spsSeriesRLCBranchLib/Series RLC Branch  LConnTagsString=__new0  RConnTagsString=__new0  BranchType=RL  Resistance=R5L  Inductance=X5L/100/pi  SetiL0=off  InitialCurrent=0  Capacitance=1e-6  Setx0=off  InitialVoltage=0  Measurements=None
  Series RLC Branch70 : spsSeriesRLCBranchLib/Series RLC Branch  LConnTagsString=__new0  RConnTagsString=__new0  BranchType=RL  Resistance=R5L  Inductance=X5L/100/pi  SetiL0=off  InitialCurrent=0  Capacitance=1e-6  Setx0=off  InitialVoltage=0  Measurements=None
  Series RLC Branch71 : spsSeriesRLCBranchLib/Series RLC Branch  LConnTagsString=__new0  RConnTagsString=__new0  BranchType=RL  Resistance=R6L  Inductance=X6L/100/pi  SetiL0=off  InitialCurrent=0  Capacitance=1e-6  Setx0=off  InitialVoltage=0  Measurements=None
  Series RLC Branch72 : spsSeriesRLCBranchLib/Series RLC Branch  LConnTagsString=__new0  RConnTagsString=__new0  BranchType=RL  Resistance=R6L  Inductance=X6L/100/pi  SetiL0=off  InitialCurrent=0  Capacitance=1e-6  Setx0=off  InitialVoltage=0  Measurements=None
  Series RLC Branch73 : spsSeriesRLCBranchLib/Series RLC Branch  LConnTagsString=__new0  RConnTagsString=__new0  BranchType=RL  Resistance=R6L  Inductance=X6L/100/pi  SetiL0=off  InitialCurrent=0  Capacitance=1e-6  Setx0=off  InitialVoltage=0  Measurements=None
  Series RLC Branch74 : spsSeriesRLCBranchLib/Series RLC Branch  LConnTagsString=__new0  RConnTagsString=__new0  BranchType=RL  Resistance=R7L  Inductance=X7L/100/pi  SetiL0=off  InitialCurrent=0  Capacitance=1e-6  Setx0=off  InitialVoltage=0  Measurements=None
  Series RLC Branch75 : spsSeriesRLCBranchLib/Series RLC Branch  LConnTagsString=__new0  RConnTagsString=__new0  BranchType=RL  Resistance=R7L  Inductance=X7L/100/pi  SetiL0=off  InitialCurrent=0  Capacitance=1e-6  Setx0=off  InitialVoltage=0  Measurements=None
  Series RLC Branch76 : spsSeriesRLCBranchLib/Series RLC Branch  LConnTagsString=__new0  RConnTagsString=__new0  BranchType=RL  Resistance=R7L  Inductance=X7L/100/pi  SetiL0=off  InitialCurrent=0  Capacitance=1e-6  Setx0=off  InitialVoltage=0  Measurements=None
  Series RLC Branch77 : spsSeriesRLCBranchLib/Series RLC Branch  LConnTagsString=__new0  RConnTagsString=__new0  BranchType=RL  Resistance=R10L  Inductance=X10L/100/pi  SetiL0=off  InitialCurrent=0  Capacitance=1e-6  Setx0=off  InitialVoltage=0  Measurements=None
  Series RLC Branch78 : spsSeriesRLCBranchLib/Series RLC Branch  LConnTagsString=__new0  RConnTagsString=__new0  BranchType=RL  Resistance=R10L  Inductance=X10L/100/pi  SetiL0=off  InitialCurrent=0  Capacitance=1e-6  Setx0=off  InitialVoltage=0  Measurements=None
  Series RLC Branch79 : spsSeriesRLCBranchLib/Series RLC Branch  LConnTagsString=__new0  RConnTagsString=__new0  BranchType=RL  Resistance=R10L  Inductance=X10L/100/pi  SetiL0=off  InitialCurrent=0  Capacitance=1e-6  Setx0=off  InitialVoltage=0  Measurements=None
  Series RLC Branch80 : spsSeriesRLCBranchLib/Series RLC Branch  LConnTagsString=__new0  RConnTagsString=__new0  BranchType=RL  Resistance=R13L  Inductance=X13L/100/pi  SetiL0=off  InitialCurrent=0  Capacitance=1e-6  Setx0=off  InitialVoltage=0  Measurements=None
  Series RLC Branch81 : spsSeriesRLCBranchLib/Series RLC Branch  LConnTagsString=__new0  RConnTagsString=__new0  BranchType=RL  Resistance=R13L  Inductance=X13L/100/pi  SetiL0=off  InitialCurrent=0  Capacitance=1e-6  Setx0=off  InitialVoltage=0  Measurements=None
  Series RLC Branch82 : spsSeriesRLCBranchLib/Series RLC Branch  LConnTagsString=__new0  RConnTagsString=__new0  BranchType=RL  Resistance=R13L  Inductance=X13L/100/pi  SetiL0=off  InitialCurrent=0  Capacitance=1e-6  Setx0=off  InitialVoltage=0  Measurements=None
  Series RLC Branch83 : spsSeriesRLCBranchLib/Series RLC Branch  LConnTagsString=__new0  RConnTagsString=__new0  BranchType=RL  Resistance=R14L  Inductance=X14L/100/pi  SetiL0=off  InitialCurrent=0  Capacitance=1e-6  Setx0=off  InitialVoltage=0  Measurements=None
  Series RLC Branch84 : spsSeriesRLCBranchLib/Series RLC Branch  LConnTagsString=__new0  RConnTagsString=__new0  BranchType=RL  Resistance=R14L  Inductance=X14L/100/pi  SetiL0=off  InitialCurrent=0  Capacitance=1e-6  Setx0=off  InitialVoltage=0  Measurements=None
  Series RLC Branch85 : spsSeriesRLCBranchLib/Series RLC Branch  LConnTagsString=__new0  RConnTagsString=__new0  BranchType=RL  Resistance=R14L  Inductance=X14L/100/pi  SetiL0=off  InitialCurrent=0  Capacitance=1e-6  Setx0=off  InitialVoltage=0  Measurements=None
  Series RLC Branch86 : spsSeriesRLCBranchLib/Series RLC Branch  LConnTagsString=__new0  RConnTagsString=__new0  BranchType=RL  Resistance=R16L  Inductance=X16L/100/pi  SetiL0=off  InitialCurrent=0  Capacitance=1e-6  Setx0=off  InitialVoltage=0  Measurements=None
  Series RLC Branch87 : spsSeriesRLCBranchLib/Series RLC Branch  LConnTagsString=__new0  RConnTagsString=__new0  BranchType=RL  Resistance=R16L  Inductance=X16L/100/pi  SetiL0=off  InitialCurrent=0  Capacitance=1e-6  Setx0=off  InitialVoltage=0  Measurements=None
  Series RLC Branch88 : spsSeriesRLCBranchLib/Series RLC Branch  LConnTagsString=__new0  RConnTagsString=__new0  BranchType=RL  Resistance=R16L  Inductance=X16L/100/pi  SetiL0=off  InitialCurrent=0  Capacitance=1e-6  Setx0=off  InitialVoltage=0  Measurements=None
  Series RLC Branch89 : spsSeriesRLCBranchLib/Series RLC Branch  LConnTagsString=__new0  RConnTagsString=__new0  BranchType=RL  Resistance=R20L  Inductance=X20L/100/pi  SetiL0=off  InitialCurrent=0  Capacitance=1e-6  Setx0=off  InitialVoltage=0  Measurements=None
  Series RLC Branch90 : spsSeriesRLCBranchLib/Series RLC Branch  LConnTagsString=__new0  RConnTagsString=__new0  BranchType=RL  Resistance=R20L  Inductance=X20L/100/pi  SetiL0=off  InitialCurrent=0  Capacitance=1e-6  Setx0=off  InitialVoltage=0  Measurements=None
  Series RLC Branch91 : spsSeriesRLCBranchLib/Series RLC Branch  LConnTagsString=__new0  RConnTagsString=__new0  BranchType=RL  Resistance=R20L  Inductance=X20L/100/pi  SetiL0=off  InitialCurrent=0  Capacitance=1e-6  Setx0=off  InitialVoltage=0  Measurements=None
  Series RLC Branch92 : spsSeriesRLCBranchLib/Series RLC Branch  LConnTagsString=__new0  RConnTagsString=__new0  BranchType=RL  Resistance=R17L  Inductance=X17L/100/pi  SetiL0=off  InitialCurrent=0  Capacitance=1e-6  Setx0=off  InitialVoltage=0  Measurements=None
  Series RLC Branch93 : spsSeriesRLCBranchLib/Series RLC Branch  LConnTagsString=__new0  RConnTagsString=__new0  BranchType=RL  Resistance=R17L  Inductance=X17L/100/pi  SetiL0=off  InitialCurrent=0  Capacitance=1e-6  Setx0=off  InitialVoltage=0  Measurements=None
  Series RLC Branch94 : spsSeriesRLCBranchLib/Series RLC Branch  LConnTagsString=__new0  RConnTagsString=__new0  BranchType=RL  Resistance=R17L  Inductance=X17L/100/pi  SetiL0=off  InitialCurrent=0  Capacitance=1e-6  Setx0=off  InitialVoltage=0  Measurements=None
  Series RLC Branch95 : spsSeriesRLCBranchLib/Series RLC Branch  LConnTagsString=__new0  RConnTagsString=__new0  BranchType=RL  Resistance=R18L  Inductance=X18L/100/pi  SetiL0=off  InitialCurrent=0  Capacitance=1e-6  Setx0=off  InitialVoltage=0  Measurements=None
  Series RLC Branch96 : spsSeriesRLCBranchLib/Series RLC Branch  LConnTagsString=__new0  RConnTagsString=__new0  BranchType=RL  Resistance=R18L  Inductance=X18L/100/pi  SetiL0=off  InitialCurrent=0  Capacitance=1e-6  Setx0=off  InitialVoltage=0  Measurements=None
  Series RLC Branch97 : spsSeriesRLCBranchLib/Series RLC Branch  LConnTagsString=__new0  RConnTagsString=__new0  BranchType=RL  Resistance=R18L  Inductance=X18L/100/pi  SetiL0=off  InitialCurrent=0  Capacitance=1e-6  Setx0=off  InitialVoltage=0  Measurements=None
  Series RLC Branch98 : spsSeriesRLCBranchLib/Series RLC Branch  LConnTagsString=__new0  RConnTagsString=__new0  BranchType=RL  Resistance=R19L  Inductance=X19L/100/pi  SetiL0=off  InitialCurrent=0  Capacitance=1e-6  Setx0=off  InitialVoltage=0  Measurements=None
  Series RLC Branch99 : spsSeriesRLCBranchLib/Series RLC Branch  LConnTagsString=__new0  RConnTagsString=__new0  BranchType=RL  Resistance=R19L  Inductance=X19L/100/pi  SetiL0=off  InitialCurrent=0  Capacitance=1e-6  Setx0=off  InitialVoltage=0  Measurements=None
  Subsystem1 : Subsystem
  Subsystem10 : Subsystem
  Switch{,1..35} (36 alike) : Switch  Criteria=u2 > Threshold  Threshold=sw  SaturateOnIntegerOverflow=off  InputSameDT=off
  T_n1 : MATLAB Function  Commented=on  TreatAsAtomicUnit=on
  T_n7 : MATLAB Function  Commented=on  TreatAsAtomicUnit=on
  T_p1 : MATLAB Function  Commented=on  TreatAsAtomicUnit=on
  T_p7 : MATLAB Function  Commented=on  TreatAsAtomicUnit=on
  Trigonometric Function{,1..3} (4 alike) : Trigonometry  Commented=on  Operator=atan2
  V1dp : Constant  Commented=on  Value=300.89
  V1qp : Constant  Commented=on  Value=8.4045
  powergui1 : spspowerguiLib/powergui  Priority=1  SimulationMode=Discrete  SampleTime=1e-5  frequency=60  Iterations=50  frequencyindice=0  Pbase=100e6  ErrMax=1e-4  UnitsV=kV  UnitsW=MW  buscounter=0  FunctionMessages=off  echomessages=off  EnableUseOfTLC=off  CurrentSourceSwitches=off  DisableSnubberDevices=off  DisableRonSwitches=off  DisableVfSwitches=off  DisplayEquations=off  AutomaticDiscreteSolvers=off  SolverType=Tustin/Backward Euler (TBE)  Interpol=off  ExternalGateDelay=off  methode=off  Ts=100  x0status=blocks  SPID=off  SwTol=0  HookPort=off  NonlinearTolerance=1e-4  nMaxIteration=100  ContinueOnMaxIteration=off  RestoreLinks=warning  ResistiveCurrentMeasurement=off  Frange=[0:2:500]  Ylog=off  Xlog=on  ShowGrid=off  save=off  variable=ZData  structure=ScopeData2  ZoomFFT=off  StartTime=0.91  cycles=4  DisplayStyle=1  fundamental=50  FreqAxis=off  MaxFrequency=1000  frequencyindicesteady=1  RmsSteady=1  display=off
  z{1..23} (23 alike) : spsSeriesRLCBranchLib/Series RLC Branch  LConnTagsString=__new0  RConnTagsString=__new0  BranchType=RL  Resistance=R  Inductance=L  SetiL0=off  InitialCurrent=0  Capacitance=1e-6  Setx0=off  InitialVoltage=0  Measurements=None
  电网电压正负序分离 : Subsystem
  tag scope: I10dn_ref=global, I10dp_ref=global, I10qn_ref=global, I10qp_ref=global, I11dn_ref=global, I11dp_ref=global, I11qn_ref=global, I11qp_ref=global, I12dn_ref=global, I12dp_ref=global, I12qn_ref=global, I12qp_ref=global, I16dn_ref=global, I16dp_ref=global, I16qn_ref=global, I16qp_ref=global, I21dn_ref=global, I21dp_ref=global, I21qn_ref=global, I21qp_ref=global, I22dn_ref=global, I22dp_ref=global, I22qn_ref=global, I22qp_ref=global, I23dn_ref=global, I23dp_ref=global, I23qn_ref=global, I23qp_ref=global, I4dn_ref=global, I4dp_ref=global, I4qn_ref=global, I4qp_ref=global, I8dn_ref=global, I8dp_ref=global, I8qn_ref=global, I8qp_ref=global, Igabc=global, Vgabc=global
  wires:
  Bus 0/1 -> [Vgabc]
  [Igabc] -> Scope10/2  "Igabc"
  [Vgabc] -> Scope10/1  "Vgabc"
  [Vgabc] -> "Power (3ph, Instantaneous)"/1
  [Igabc] -> "Power (3ph, Instantaneous)"/2
  "Power (3ph, Instantaneous)"/1 -> Scope8/1  "P"
  "Power (3ph, Instantaneous)"/2 -> Scope8/2  "Q"
  Bus 0/2 -> [Igabc]
  [V4] -> "Power (3ph, Instantaneous)1"/1, Scope7/1  "V1"
  [I4] -> "Power (3ph, Instantaneous)1"/2, Scope7/2  "I1"
  [UVF4] -> Demux/1
  Demux/1 -> Scope1/1  "Vp"
  Demux/2 -> Scope1/2  "Vn"
  Demux/3 -> Scope1/3  "VUF"
  Demux1/1 -> Scope4/1
  Demux1/2 -> Scope4/2
  Demux1/3 -> Scope4/3
  [UVF8] -> Demux1/1
  [I8] -> "Power (3ph, Instantaneous)2"/2, Scope/2
  [V8] -> "Power (3ph, Instantaneous)2"/1, Scope/1  "V7"
  [PQ8] -> Demux3/1  "PQ"
  [PQ4] -> Gain2/1  "PQ"
  Demux2/2 -> Scope2/2  "Q"
  Constant1/1 -> Trigonometric Function/1
  [Vgabc] -> 电网电压正负序分离/1(In1)
  Trigonometric Function/1 -> T_p1/3(ph)
  Constant/1 -> Trigonometric Function/2
  Constant2/1 -> Switch/1
  Constant3/1 -> Switch1/1
  Constant4/1 -> Trigonometric Function1/2
  Trigonometric Function1/1 -> T_p7/3(ph)
  Constant5/1 -> Trigonometric Function1/1
  V1dp/1 -> Trigonometric Function2/2
  V1qp/1 -> Trigonometric Function2/1
  Constant13/1 -> Trigonometric Function3/1
  Constant12/1 -> Trigonometric Function3/2
  电网电压正负序分离/1(vcd_p) -> Scope9/1
  电网电压正负序分离/2(vcq_p) -> Scope9/2
  电网电压正负序分离/3(vcd_n) -> Scope9/3
  电网电压正负序分离/4(vcq_n) -> Scope9/4
  Trigonometric Function2/1 -> Gain/1
  Trigonometric Function3/1 -> Gain1/1
  Gain/1 -> T_n1/3(ph)
  Gain1/1 -> T_n7/3(ph)
  Clock/1 -> Switch/2
  Constant8/1 -> Switch/3
  Switch/1 -> [I4dp_ref]
  Switch1/1 -> [I4qp_ref]
  Constant9/1 -> Switch1/3
  Clock1/1 -> Switch1/2
  Clock2/1 -> Switch2/2
  Constant16/1 -> Switch2/3
  Constant17/1 -> Switch3/3
  Clock3/1 -> Switch3/2
  Clock7/1 -> Switch7/2
  Constant19/1 -> Switch7/3
  Constant18/1 -> Switch6/3
  Clock6/1 -> Switch6/2
  Clock5/1 -> Switch5/2
  Constant21/1 -> Switch5/3
  Constant20/1 -> Switch4/3
  Clock4/1 -> Switch4/2
  Demux3/1 -> Scope6/1  "P"
  Demux3/2 -> Scope6/2  "Q"
  "Power (3ph, Instantaneous)2"/1 -> Scope12/1  "P"
  "Power (3ph, Instantaneous)2"/2 -> Scope12/2  "Q"
  "Power (3ph, Instantaneous)1"/1 -> Scope11/1  "P"
  "Power (3ph, Instantaneous)1"/2 -> Scope11/2  "Q"
  Constant10/1 -> Switch2/1
  Constant11/1 -> Switch3/1
  Constant6/1 -> Switch4/1
  Constant7/1 -> Switch5/1
  Constant14/1 -> Switch6/1
  Constant15/1 -> Switch7/1
  Switch2/1 -> [I4dn_ref]
  Switch3/1 -> [I4qn_ref]
  Switch6/1 -> [I8dn_ref]
  Switch7/1 -> [I8qn_ref]
  Switch4/1 -> [I8dp_ref]
  Switch5/1 -> [I8qp_ref]
  Demux4/3 -> Scope3/3  "VUF"
  "Power (3ph, Instantaneous)3"/2 -> Scope5/2  "Q"
  Demux4/1 -> Scope3/1  "Vp"
  [V10] -> "Power (3ph, Instantaneous)3"/1, Scope14/1  "V1"
  [PQ10] -> Demux5/1  "PQ"
  Demux5/1 -> Scope13/1  "P"
  [UVF10] -> Demux4/1
  Demux5/2 -> Scope13/2  "Q"
  Demux4/2 -> Scope3/2  "Vn"
  "Power (3ph, Instantaneous)3"/1 -> Scope5/1  "P"
  [I10] -> "Power (3ph, Instantaneous)3"/2, Scope14/2  "I1"
  Demux6/3 -> Scope15/3  "VUF"
  "Power (3ph, Instantaneous)4"/2 -> Scope16/2  "Q"
  Demux6/1 -> Scope15/1  "Vp"
  [V11] -> "Power (3ph, Instantaneous)4"/1, Scope18/1  "V1"
  [PQ11] -> Demux7/1  "PQ"
  Demux7/1 -> Scope17/1  "P"
  [UVF11] -> Demux6/1
  Demux7/2 -> Scope17/2  "Q"
  Demux6/2 -> Scope15/2  "Vn"
  "Power (3ph, Instantaneous)4"/1 -> Scope16/1  "P"
  [I11] -> "Power (3ph, Instantaneous)4"/2, Scope18/2  "I1"
  Demux8/3 -> Scope19/3  "VUF"
  "Power (3ph, Instantaneous)5"/2 -> Scope20/2  "Q"
  Demux8/1 -> Scope19/1  "Vp"
  [V12] -> "Power (3ph, Instantaneous)5"/1, Scope22/1  "V1"
  [PQ12] -> Demux9/1  "PQ"
  Demux9/1 -> Scope21/1  "P"
  [UVF12] -> Demux8/1
  Demux9/2 -> Scope21/2  "Q"
  Demux8/2 -> Scope19/2  "Vn"
  "Power (3ph, Instantaneous)5"/1 -> Scope20/1  "P"
  [I12] -> "Power (3ph, Instantaneous)5"/2, Scope22/2  "I1"
  Demux10/3 -> Scope23/3  "VUF"
  "Power (3ph, Instantaneous)6"/2 -> Scope24/2  "Q"
  Demux10/1 -> Scope23/1  "Vp"
  [V16] -> Scope26/1, "Power (3ph, Instantaneous)6"/1  "V1"
  [PQ16] -> Demux11/1  "PQ"
  Demux11/1 -> Scope25/1  "P"
  [UVF16] -> Demux10/1
  Demux11/2 -> Scope25/2  "Q"
  Demux10/2 -> Scope23/2  "Vn"
  "Power (3ph, Instantaneous)6"/1 -> Scope24/1  "P"
  [I16] -> Scope26/2, "Power (3ph, Instantaneous)6"/2  "I1"
  Demux12/3 -> Scope27/3  "VUF"
  "Power (3ph, Instantaneous)7"/2 -> Scope28/2  "Q"
  Demux12/1 -> Scope27/1  "Vp"
  [V23] -> "Power (3ph, Instantaneous)7"/1, Scope30/1  "V1"
  [PQ23] -> Demux13/1  "PQ"
  Demux13/1 -> Scope29/1  "P"
  [UVF23] -> Demux12/1
  Demux13/2 -> Scope29/2  "Q"
  Demux12/2 -> Scope27/2  "Vn"
  "Power (3ph, Instantaneous)7"/1 -> Scope28/1  "P"
  [I23] -> "Power (3ph, Instantaneous)7"/2, Scope30/2  "I1"
  Demux14/3 -> Scope31/3  "VUF"
  "Power (3ph, Instantaneous)8"/2 -> Scope32/2  "Q"
  Demux14/1 -> Scope31/1  "Vp"
  [V21] -> "Power (3ph, Instantaneous)8"/1, Scope34/1  "V1"
  [PQ21] -> Demux15/1  "PQ"
  Demux15/1 -> Scope33/1  "P"
  [UVF21] -> Demux14/1
  Demux15/2 -> Scope33/2  "Q"
  Demux14/2 -> Scope31/2  "Vn"
  "Power (3ph, Instantaneous)8"/1 -> Scope32/1  "P"
  [I21] -> Scope34/2, "Power (3ph, Instantaneous)8"/2  "I1"
  Demux16/3 -> Scope35/3  "VUF"
  "Power (3ph, Instantaneous)9"/2 -> Scope36/2  "Q"
  Demux16/1 -> Scope35/1  "Vp"
  [V22] -> "Power (3ph, Instantaneous)9"/1, Scope38/1  "V1"
  [PQ22] -> Demux17/1  "PQ"
  Demux17/1 -> Scope37/1  "P"
  [UVF22] -> Demux16/1
  Demux17/2 -> Scope37/2  "Q"
  Demux16/2 -> Scope35/2  "Vn"
  "Power (3ph, Instantaneous)9"/1 -> Scope36/1  "P"
  [I22] -> "Power (3ph, Instantaneous)9"/2, Scope38/2  "I1"
  Gain2/1 -> Demux2/1
  Demux2/1 -> Scope2/1  "P"
  Constant57/1 -> Switch9/1
  Constant56/1 -> Switch8/1
  Clock8/1 -> Switch8/2
  Constant50/1 -> Switch8/3
  Constant51/1 -> Switch9/3
  Clock9/1 -> Switch9/2
  Clock11/1 -> Switch11/2
  Constant53/1 -> Switch11/3
  Constant52/1 -> Switch10/3
  Clock10/1 -> Switch10/2
  Constant54/1 -> Switch10/1
  Constant55/1 -> Switch11/1
  Switch8/1 -> [I21dp_ref]
  Switch9/1 -> [I21qp_ref]
  Switch10/1 -> [I21dn_ref]
  Switch11/1 -> [I21qn_ref]
  Clock12/1 -> Switch15/2, Switch14/2, Switch13/2, Switch12/2
  Constant28/1 -> Switch12/1
  Switch12/1 -> [I10dp_ref]
  Constant29/1 -> Switch13/1
  Switch13/1 -> [I10qp_ref]
  Switch14/1 -> [I10dn_ref]
  Switch15/1 -> [I10qn_ref]
  Constant22/1 -> Switch14/1
  Constant23/1 -> Switch15/1
  Constant38/1 -> Switch13/3, Switch14/3, Switch15/3
  Constant39/1 -> Switch12/3
  Constant41/1 -> Switch16/3
  Constant40/1 -> Switch19/3, Switch18/3, Switch17/3
  Constant25/1 -> Switch19/1
  Constant24/1 -> Switch18/1
  Switch19/1 -> [I11qn_ref]
  Switch18/1 -> [I11dn_ref]
  Switch17/1 -> [I11qp_ref]
  Constant27/1 -> Switch17/1
  Switch16/1 -> [I11dp_ref]
  Constant26/1 -> Switch16/1
  Clock13/1 -> Switch16/2, Switch17/2, Switch18/2, Switch19/2
  Clock14/1 -> Switch23/2, Switch22/2, Switch21/2, Switch20/2
  Constant32/1 -> Switch20/1
  Switch20/1 -> [I12dp_ref]
  Constant33/1 -> Switch21/1
  Switch21/1 -> [I12qp_ref]
  Switch22/1 -> [I12dn_ref]
  Switch23/1 -> [I12qn_ref]
  Constant30/1 -> Switch22/1
  Constant31/1 -> Switch23/1
  Constant58/1 -> Switch21/3, Switch22/3, Switch23/3
  Constant59/1 -> Switch20/3
  Constant61/1 -> Switch24/3
  Constant60/1 -> Switch27/3, Switch26/3, Switch25/3
  Constant35/1 -> Switch27/1
  Constant34/1 -> Switch26/1
  Switch27/1 -> [I16qn_ref]
  Switch26/1 -> [I16dn_ref]
  Switch25/1 -> [I16qp_ref]
  Constant37/1 -> Switch25/1
  Switch24/1 -> [I16dp_ref]
  Constant36/1 -> Switch24/1
  Clock15/1 -> Switch24/2, Switch25/2, Switch26/2, Switch27/2
  Clock16/1 -> Switch31/2, Switch30/2, Switch29/2, Switch28/2
  Constant44/1 -> Switch28/1
  Switch28/1 -> [I22dp_ref]
  Constant45/1 -> Switch29/1
  Switch29/1 -> [I22qp_ref]
  Switch30/1 -> [I22dn_ref]
  Constant42/1 -> Switch30/1
  Constant43/1 -> Switch31/1
  Constant62/1 -> Switch29/3, Switch30/3, Switch31/3
  Constant63/1 -> Switch28/3
  Switch31/1 -> [I22qn_ref]
  Constant65/1 -> Switch32/3
  Constant64/1 -> Switch35/3, Switch34/3, Switch33/3
  Constant47/1 -> Switch35/1
  Constant46/1 -> Switch34/1
  Constant49/1 -> Switch33/1
  Constant48/1 -> Switch32/1
  Clock17/1 -> Switch32/2, Switch33/2, Switch34/2, Switch35/2
  Switch32/1 -> [I23dp_ref]
  Switch33/1 -> [I23qp_ref]
  Switch34/1 -> [I23dn_ref]
  Switch35/1 -> [I23qn_ref]
  [I_load8] -> "Power (3ph, Instantaneous)10"/2
  Subsystem10/2(O2) -> Mux10/2
  Subsystem10/1(O1) -> Mux10/1
  Subsystem10/3(O3) -> Mux10/3
  Mux10/1 -> [I_load8]
  Mux1/1 -> [I_load11]
  Subsystem1/3(O3) -> Mux1/3
  Subsystem1/1(O1) -> Mux1/1
  Subsystem1/2(O2) -> Mux1/2
  [I_load11] -> "Power (3ph, Instantaneous)12"/2
  [I_load3] -> "Power (3ph, Instantaneous)13"/2
  [V13] -> IBR1输出电压正负序分离/1(In1), Scope43/1  "V1"
  [I13] -> Scope43/2  "I1"
  [V8] -> "Power (3ph, Instantaneous)10"/1  "V7"
  "Power (3ph, Instantaneous)10"/1 -> Scope39/1  "P"
  "Power (3ph, Instantaneous)10"/2 -> Scope39/2  "Q"
  [V11] -> "Power (3ph, Instantaneous)12"/1  "V1"
  "Power (3ph, Instantaneous)12"/1 -> Scope40/1  "P"
  "Power (3ph, Instantaneous)12"/2 -> Scope40/2  "Q"
  [V14] -> "Power (3ph, Instantaneous)13"/1  "V1"
  "Power (3ph, Instantaneous)13"/1 -> Scope41/1  "P"
  "Power (3ph, Instantaneous)13"/2 -> Scope41/2  "Q"
  IBR1输出电压正负序分离/4(vcq_n) -> IBR2/4(vcq_n)
  IBR2/2(Vc_n) -> Scope44/2  "Vn"
  IBR1输出电压正负序分离/2(vcq_p) -> IBR2/2(vcq_p)
  IBR1输出电压正负序分离/3(vcd_n) -> IBR2/3(vcd_n)
  IBR2/1(Vc_p) -> Scope44/1  "Vp"
  IBR2/3(VUF) -> Scope44/3  "VUF"
  IBR1输出电压正负序分离/1(vcd_p) -> IBR2/1(vcd_p)
  IBR1/3(VUF) -> Scope46/3  "VUF"
  IBR1/1(Vc_p) -> Scope46/1  "Vp"
  IBR1输出电压正负序分离1/3(vcd_n) -> IBR1/3(vcd_n)
  IBR1输出电压正负序分离1/2(vcq_p) -> IBR1/2(vcq_p)
  IBR1/2(Vc_n) -> Scope46/2  "Vn"
  IBR1输出电压正负序分离1/4(vcq_n) -> IBR1/4(vcq_n)
  [I1] -> Scope45/2  "I1"
  [V1] -> Scope45/1, IBR1输出电压正负序分离1/1(In1)  "V1"
  IBR1输出电压正负序分离1/1(vcd_p) -> IBR1/1(vcd_p)
  connections:
  Bus 1/RConn1 -- Series RLC Branch3/RConn1
  Bus 1/RConn2 -- Series RLC Branch4/RConn1
  Bus 1/RConn3 -- z1/RConn1
  Grid/RConn1 -- Bus 0/RConn1
  Grid/RConn2 -- Bus 0/RConn2
  Grid/RConn3 -- Bus 0/RConn3
  Series RLC Branch5/LConn1 -- Bus 1/LConn1
  Bus 1/LConn3 -- z2/LConn1
  Bus 0/LConn1 -- Series RLC Branch3/LConn1
  Bus 0/LConn2 -- Series RLC Branch4/LConn1
  Bus 0/LConn3 -- z1/LConn1
  z4/LConn1 -- Bus 3/LConn3
  Bus 3/RConn3 -- Series RLC Branch58/LConn1 -- z3/RConn1
  Series RLC Branch10/LConn1 -- Bus 3/LConn2
  Bus 3/RConn2 -- Series RLC Branch57/LConn1 -- Series RLC Branch8/RConn1
  Bus 3/RConn1 -- Series RLC Branch56/LConn1 -- Series RLC Branch7/RConn1
  Series RLC Branch9/LConn1 -- Bus 3/LConn1
  z5/LConn1 -- Bus 4/RConn3 -- Series RLC Branch67/LConn1 -- z4/RConn1
  Series RLC Branch12/LConn1 -- Bus 4/RConn1 -- Series RLC Branch65/LConn1 -- Series RLC Branch9/RConn1
  Series RLC Branch11/LConn1 -- Bus 4/RConn2 -- Series RLC Branch66/LConn1 -- Series RLC Branch10/RConn1
  Bus 5/RConn2 -- Series RLC Branch69/RConn1 -- Series RLC Branch11/RConn1
  Bus 5/RConn3 -- Series RLC Branch70/RConn1 -- z5/RConn1
  Bus 5/RConn1 -- Series RLC Branch68/RConn1 -- Series RLC Branch12/RConn1
  Series RLC Branch5/RConn1 -- Bus 2/RConn1
  Series RLC Branch6/RConn1 -- Bus 2/RConn2
  z2/RConn1 -- Bus 2/RConn3
  Bus 1/LConn2 -- Series RLC Branch6/LConn1
  Series RLC Branch7/LConn1 -- Series RLC Branch33/LConn1 -- Bus 2/LConn1 -- Series RLC Branch49/LConn1
  Series RLC Branch8/LConn1 -- Series RLC Branch34/LConn1 -- Bus 2/LConn2 -- Series RLC Branch50/LConn1
  z3/LConn1 -- z13/LConn1 -- Bus 2/LConn3 -- Series RLC Branch55/LConn1
  Bus 9/RConn1 -- Series RLC Branch23/RConn1
  Bus 9/RConn2 -- Series RLC Branch24/RConn1
  Bus 9/RConn3 -- z9/RConn1
  Bus 10/RConn3 -- z10/RConn1 -- Series RLC Branch79/LConn1
  Bus 10/RConn2 -- Series RLC Branch78/LConn1 -- Series RLC Branch26/RConn1
  Series RLC Branch25/RConn1 -- Series RLC Branch77/LConn1 -- Bus 10/RConn1
  z8/LConn1 -- Bus 7/LConn3
  z8/RConn1 -- Subsystem10/LConn3 -- Bus 8/RConn3
  Bus 5/LConn2 -- Series RLC Branch16/RConn1 -- Series RLC Branch24/LConn1
  Bus 5/LConn1 -- z6/RConn1 -- Series RLC Branch23/LConn1
  Series RLC Branch25/LConn1 -- Series RLC Branch29/LConn1 -- Series RLC Branch27/LConn1 -- Bus 9/LConn1
  Series RLC Branch26/LConn1 -- Series RLC Branch30/LConn1 -- Series RLC Branch28/LConn1 -- Bus 9/LConn2
  z10/LConn1 -- z12/LConn1 -- z11/LConn1 -- Bus 9/LConn3
  Bus 11/RConn1 -- Subsystem1/LConn1 -- Series RLC Branch27/RConn1
  Bus 11/RConn2 -- Subsystem1/LConn2 -- Series RLC Branch28/RConn1
  Bus 11/RConn3 -- z11/RConn1 -- Subsystem1/LConn3
  Bus 12/RConn1 -- Series RLC Branch29/RConn1
  Bus 12/RConn2 -- Series RLC Branch30/RConn1
  Bus 12/RConn3 -- z12/RConn1
  Bus 6/LConn1 -- Series RLC Branch19/LConn1
  Bus 6/LConn2 -- Series RLC Branch20/LConn1
  Bus 6/LConn3 -- z7/LConn1
  Bus 7/LConn1 -- Series RLC Branch21/LConn1
  Bus 7/LConn2 -- Series RLC Branch22/LConn1
  Bus 7/RConn1 -- Series RLC Branch74/RConn1 -- Series RLC Branch19/RConn1
  Bus 7/RConn2 -- Series RLC Branch75/RConn1 -- Series RLC Branch20/RConn1
  Bus 7/RConn3 -- Series RLC Branch76/RConn1 -- z7/RConn1
  Bus 6/RConn1 -- z6/LConn1 -- Series RLC Branch71/RConn1
  Bus 6/RConn2 -- Series RLC Branch72/RConn1 -- Series RLC Branch16/LConn1
  Bus 6/RConn3 -- Series RLC Branch73/RConn1 -- Series RLC Branch15/LConn1
  Bus 13/RConn1 -- Series RLC Branch80/RConn1 -- Series RLC Branch33/RConn1
  Bus 13/RConn2 -- Series RLC Branch81/RConn1 -- Series RLC Branch34/RConn1
  Bus 13/RConn3 -- z13/RConn1 -- Series RLC Branch82/RConn1
  Bus 14/LConn1 -- Series RLC Branch37/LConn1 -- Series RLC Branch45/LConn1
  Bus 14/LConn2 -- Series RLC Branch38/LConn1 -- Series RLC Branch46/LConn1
  Bus 14/LConn3 -- z15/LConn1 -- z17/LConn1
  Bus 14/RConn1 -- Series RLC Branch83/RConn1 -- Series RLC Branch35/RConn1
  Bus 14/RConn2 -- Series RLC Branch84/RConn1 -- Series RLC Branch36/RConn1
  Bus 14/RConn3 -- Series RLC Branch85/RConn1 -- z14/RConn1
  Bus 13/LConn1 -- Series RLC Branch35/LConn1
  Bus 13/LConn2 -- Series RLC Branch36/LConn1
  Bus 13/LConn3 -- z14/LConn1
  Bus 15/RConn1 -- Series RLC Branch32/RConn1 -- Series RLC Branch37/RConn1
  Bus 15/RConn2 -- Series RLC Branch38/RConn1 -- Series RLC Branch31/RConn1
  Bus 15/RConn3 -- Series RLC Branch41/RConn1 -- z15/RConn1
  Bus 15/LConn1 -- Series RLC Branch39/LConn1
  Bus 15/LConn2 -- Series RLC Branch40/LConn1
  Bus 15/LConn3 -- z16/LConn1
  Bus 16/RConn1 -- Series RLC Branch86/RConn1 -- Series RLC Branch39/RConn1
  Bus 16/RConn2 -- Series RLC Branch87/RConn1 -- Series RLC Branch40/RConn1
  Bus 16/RConn3 -- Series RLC Branch88/RConn1 -- z16/RConn1
  Bus 17/RConn1 -- Series RLC Branch92/RConn1 -- Series RLC Branch45/RConn1
  Bus 17/RConn2 -- Series RLC Branch46/RConn1 -- Series RLC Branch93/RConn1
  Bus 17/RConn3 -- Series RLC Branch94/RConn1 -- z17/RConn1
  Bus 18/RConn3 -- Series RLC Branch97/RConn1 -- z18/RConn1
  Bus 18/RConn2 -- Series RLC Branch48/RConn1 -- Series RLC Branch96/RConn1
  Bus 18/RConn1 -- Series RLC Branch95/RConn1 -- Series RLC Branch47/RConn1
  Series RLC Branch47/LConn1 -- Series RLC Branch51/LConn1 -- Bus 17/LConn1
  Series RLC Branch48/LConn1 -- Series RLC Branch52/LConn1 -- Bus 17/LConn2
  z18/LConn1 -- z22/LConn1 -- Bus 17/LConn3
  Bus 22/RConn3 -- z22/RConn1 -- Series RLC Branch103/RConn1
  Bus 22/RConn2 -- Series RLC Branch102/RConn1 -- Series RLC Branch52/RConn1
  Bus 22/RConn1 -- Series RLC Branch51/RConn1 -- Series RLC Branch101/RConn1
  Bus 19/RConn2 -- Series RLC Branch99/RConn1 -- Series RLC Branch54/RConn1
  Bus 19/RConn1 -- Series RLC Branch53/RConn1 -- Series RLC Branch98/RConn1
  Bus 19/RConn3 -- Series RLC Branch100/RConn1 -- z19/RConn1
  Bus 18/LConn1 -- Series RLC Branch53/LConn1
  Bus 18/LConn2 -- Series RLC Branch54/LConn1
  Bus 18/LConn3 -- z19/LConn1
  Bus 20/RConn3 -- z20/RConn1 -- Series RLC Branch90/RConn1
  Bus 20/RConn1 -- Series RLC Branch89/RConn1 -- Series RLC Branch59/RConn1
  Bus 20/RConn2 -- Series RLC Branch60/RConn1 -- Series RLC Branch91/RConn1
  Bus 23/RConn2 -- Series RLC Branch105/RConn1 -- Series RLC Branch62/RConn1
  Bus 23/RConn1 -- Series RLC Branch104/RConn1 -- Series RLC Branch61/RConn1
  Bus 23/RConn3 -- Series RLC Branch106/RConn1 -- z23/RConn1
  Bus 21/RConn3 -- z21/RConn1 -- Series RLC Branch44/RConn1
  Bus 21/RConn1 -- Series RLC Branch63/RConn1 -- Series RLC Branch42/RConn1
  Series RLC Branch63/LConn1 -- Bus 20/LConn1
  Bus 20/LConn2 -- Series RLC Branch64/LConn1
  z21/LConn1 -- Bus 20/LConn3
  Series RLC Branch59/LConn1 -- Series RLC Branch61/LConn1 -- Bus 19/LConn1
  Series RLC Branch60/LConn1 -- Series RLC Branch62/LConn1 -- Bus 19/LConn2
  z20/LConn1 -- z23/LConn1 -- Bus 19/LConn3
  Series RLC Branch21/RConn1 -- Bus 8/RConn1 -- Subsystem10/LConn1
  Series RLC Branch22/RConn1 -- Bus 8/RConn2 -- Subsystem10/LConn2
  Bus 5/LConn3 -- Series RLC Branch15/RConn1 -- z9/LConn1
  Bus 8/LConn1 -- IBR-8/RConn1
  IBR-8/RConn2 -- Bus 8/LConn2
  IBR-8/RConn3 -- Bus 8/LConn3
  IBR-10/RConn1 -- Bus 10/LConn1
  IBR-10/RConn2 -- Bus 10/LConn2
  IBR-10/RConn3 -- Bus 10/LConn3
  IBR-11/RConn1 -- Bus 11/LConn1
  IBR-11/RConn2 -- Bus 11/LConn2
  IBR-11/RConn3 -- Bus 11/LConn3
  Bus 12/LConn1 -- IBR-12/RConn1
  Bus 12/LConn2 -- IBR-12/RConn2
  Bus 12/LConn3 -- IBR-12/RConn3
  IBR-16/RConn1 -- Bus 16/LConn1
  IBR-16/RConn2 -- Bus 16/LConn2
  IBR-16/RConn3 -- Bus 16/LConn3
  IBR-21/RConn1 -- Bus 21/LConn1
  IBR-21/RConn2 -- Bus 21/LConn2
  IBR-21/RConn3 -- Bus 21/LConn3
  IBR-23/RConn1 -- Bus 23/LConn1
  IBR-23/RConn2 -- Bus 23/LConn2
  IBR-23/RConn3 -- Bus 23/LConn3
  IBR-22/RConn1 -- Bus 22/LConn1
  Bus 22/LConn2 -- IBR-22/RConn2
  Bus 22/LConn3 -- IBR-22/RConn3
  Bus 4/LConn2 -- IBR4/RConn2
  Bus 4/LConn1 -- IBR4/RConn1
  Bus 4/LConn3 -- IBR4/RConn3
  Series RLC Branch1/RConn1 -- Series RLC Branch13/RConn1 -- Series RLC Branch2/RConn1
  Series RLC Branch1/LConn1 -- Subsystem10/RConn1
  Series RLC Branch13/LConn1 -- Subsystem10/RConn3
  Series RLC Branch2/LConn1 -- Subsystem10/RConn2
  Series RLC Branch14/RConn1 -- Series RLC Branch18/RConn1 -- Series RLC Branch17/RConn1
  Series RLC Branch18/LConn1 -- Subsystem1/RConn3
  Series RLC Branch14/LConn1 -- Subsystem1/RConn1
  Series RLC Branch17/LConn1 -- Subsystem1/RConn2
  Bus 21/RConn2 -- Series RLC Branch64/RConn1 -- Series RLC Branch43/RConn1
  Series RLC Branch50/RConn1 -- Series RLC Branch49/RConn1 -- Series RLC Branch55/RConn1
  Series RLC Branch56/RConn1 -- Series RLC Branch58/RConn1 -- Series RLC Branch57/RConn1
  Series RLC Branch65/RConn1 -- Series RLC Branch66/RConn1 -- Series RLC Branch67/RConn1
  Series RLC Branch68/LConn1 -- Series RLC Branch70/LConn1 -- Series RLC Branch69/LConn1
  Series RLC Branch71/LConn1 -- Series RLC Branch72/LConn1 -- Series RLC Branch73/LConn1
  Series RLC Branch74/LConn1 -- Series RLC Branch76/LConn1 -- Series RLC Branch75/LConn1
  Series RLC Branch77/RConn1 -- Series RLC Branch78/RConn1 -- Series RLC Branch79/RConn1
  Series RLC Branch80/LConn1 -- Series RLC Branch81/LConn1 -- Series RLC Branch82/LConn1
  Series RLC Branch83/LConn1 -- Series RLC Branch84/LConn1 -- Series RLC Branch85/LConn1
  Series RLC Branch32/LConn1 -- Series RLC Branch31/LConn1 -- Series RLC Branch41/LConn1
  Series RLC Branch88/LConn1 -- Series RLC Branch87/LConn1 -- Series RLC Branch86/LConn1
  Series RLC Branch42/LConn1 -- Series RLC Branch44/LConn1 -- Series RLC Branch43/LConn1
  Series RLC Branch89/LConn1 -- Series RLC Branch91/LConn1 -- Series RLC Branch90/LConn1
  Series RLC Branch92/LConn1 -- Series RLC Branch93/LConn1 -- Series RLC Branch94/LConn1
  Series RLC Branch95/LConn1 -- Series RLC Branch97/LConn1 -- Series RLC Branch96/LConn1
  Series RLC Branch98/LConn1 -- Series RLC Branch99/LConn1 -- Series RLC Branch100/LConn1
  Series RLC Branch101/LConn1 -- Series RLC Branch102/LConn1 -- Series RLC Branch103/LConn1
  Series RLC Branch104/LConn1 -- Series RLC Branch105/LConn1 -- Series RLC Branch106/LConn1
